simulink model "forward_inverse"  (R2023a)
settings: Solver=VariableStepAuto  StartTime=0.0  StopTime=1  RelTol=1e-3
settings Model: Creator=jeffk  LastModifiedBy=mluser
settings OptimizationCC: ReuseModelBlockBuffer=off

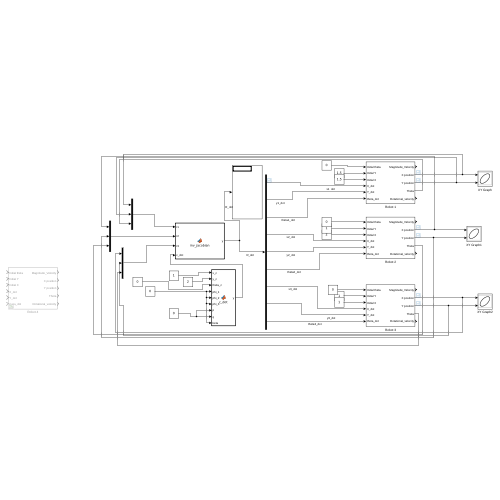
[thumbnail: Simulink's stored preview of the top-level diagram]
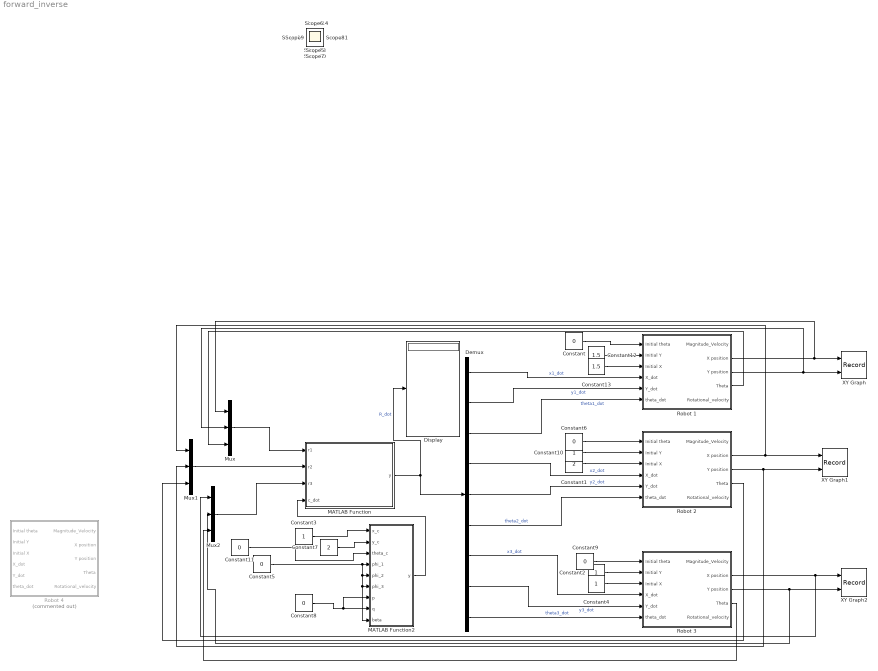
== system forward_inverse ==
  Constant{,5..6,8..9,11} (6 alike) : Constant  Value=0
  Constant1 : Constant  Value=2
  Constant{2..4,10} (4 alike) : Constant
  Constant12 : Constant  Value=1.5
  Constant13 : Constant  Value=1.5
  Constant7 : Constant  Value=2
  Demux : Demux  Outputs=9
  Display : Display
  MATLAB Function : MATLAB Function  TreatAsAtomicUnit=on
  MATLAB Function2 : MATLAB Function  TreatAsAtomicUnit=on
  Mux : Mux  Inputs=3
  Mux1 : Mux  Inputs=3
  Mux2 : Mux  Inputs=3
  Robot 1 : Subsystem
  Robot 2 : Subsystem
  Robot 3 : Subsystem
  Robot 4 : Subsystem  Commented=on
  XY Graph : Record  VariableName=robot1xy  RecordToWorkspace=on  FileSettingsInternal="{\"entries\":[{\"content\":{\"excelSettings\":{\"content\":{},\"type\":\"Streamout.ExcelSettings\"}},\"type\":\"Streamout.FileSettingStorage\",\"uuid\":\"\"}],\"packageUris\":[\"http:\\/\\/schema.mathworks.com\\/mf0\\/streamout_blocks\\/R2020a\"],\"version\":\"1.0\"}"  Layout=[1 1]  SignalsInternal="{\"entries\":[{\"content\":{\"signals\":[{\"content\":{\"blockPath\":[],\"dimensions\":[1,1],\"domain\":\"\",\"lineColor\":\"#a2142f\",\"plots\":[1],\"port\":1,\"signalID\":51,\"signalName\":\"Robot 1:2\"},\"type\":\"RecordBlkView.Signal\",\"uuid\":\"\"},{\"content\":{\"blockPath\":[],\"dimensions\":[1,1],\"domain\":\"\",\"lineColor\":\"#139fff\",\"plots\":[1],\"port\":2,\"signalID\":54,\"signalName\":\"Robot 1:3\"},\"type\":\"RecordBlkView.Signal\",\"uuid\":\"\"}]},\"type\":\"RecordBlkView.InputSignals\",\"uuid\":\"\"}],\"packageUris\":[\"http:\\/\\/schema.mathworks.com\\/mf0\\/streamout_blocks\\/R2020a\"],\"version\":\"1.0\"}"  VisualizationBindings="{\"xyplotplugin\":{\"info\":[{\"series\":[{\"bindingParametersList\":[{\"parameter\":\"X-Axis\",\"signalID\":51,\"signalName\":\"Robot 1:2\"},{\"parameter\":\"Y-Axis\",\"signalID\":54,\"signalName\":\"Robot 1:3\"}],\"seriesID\":6107}],\"subplotID\":1}]}}"  CompatibilityTag=XY
  XY Graph1 : Record  VariableName=robot2xy  RecordToWorkspace=on  FileSettingsInternal="{\"entries\":[{\"content\":{\"excelSettings\":{\"content\":{},\"type\":\"Streamout.ExcelSettings\"}},\"type\":\"Streamout.FileSettingStorage\",\"uuid\":\"\"}],\"packageUris\":[\"http:\\/\\/schema.mathworks.com\\/mf0\\/streamout_blocks\\/R2020a\"],\"version\":\"1.0\"}"  Layout=[1 1]  SignalsInternal="{\"entries\":[{\"content\":{\"signals\":[{\"content\":{\"blockPath\":[],\"dimensions\":[1,1],\"domain\":\"\",\"lineColor\":\"#a2142f\",\"plots\":[1],\"port\":1,\"signalID\":35,\"signalName\":\"Robot 2:2\"},\"type\":\"RecordBlkView.Signal\",\"uuid\":\"\"},{\"content\":{\"blockPath\":[],\"dimensions\":[1,1],\"domain\":\"\",\"lineColor\":\"#139fff\",\"plots\":[1],\"port\":2,\"signalID\":38,\"signalName\":\"Robot 2:3\"},\"type\":\"RecordBlkView.Signal\",\"uuid\":\"\"}]},\"type\":\"RecordBlkView.InputSignals\",\"uuid\":\"\"}],\"packageUris\":[\"http:\\/\\/schema.mathworks.com\\/mf0\\/streamout_blocks\\/R2020a\"],\"version\":\"1.0\"}"  VisualizationBindings="{\"xyplotplugin\":{\"info\":[{\"series\":[{\"bindingParametersList\":[{\"parameter\":\"X-Axis\",\"signalID\":35,\"signalName\":\"Robot 2:2\"},{\"parameter\":\"Y-Axis\",\"signalID\":38,\"signalName\":\"Robot 2:3\"}],\"seriesID\":14312}],\"subplotID\":1}]}}"  CompatibilityTag=XY
  XY Graph2 : Record  VariableName=robot3xy  RecordToWorkspace=on  FileSettingsInternal="{\"entries\":[{\"content\":{\"excelSettings\":{\"content\":{},\"type\":\"Streamout.ExcelSettings\"}},\"type\":\"Streamout.FileSettingStorage\",\"uuid\":\"\"}],\"packageUris\":[\"http:\\/\\/schema.mathworks.com\\/mf0\\/streamout_blocks\\/R2020a\"],\"version\":\"1.0\"}"  Layout=[1 1]  SignalsInternal="{\"entries\":[{\"content\":{\"signals\":[{\"content\":{\"blockPath\":[],\"dimensions\":[1,1],\"domain\":\"\",\"lineColor\":\"#a2142f\",\"plots\":[1],\"port\":1,\"signalID\":43,\"signalName\":\"Robot 3:2\"},\"type\":\"RecordBlkView.Signal\",\"uuid\":\"\"},{\"content\":{\"blockPath\":[],\"dimensions\":[1,1],\"domain\":\"\",\"lineColor\":\"#139fff\",\"plots\":[1],\"port\":2,\"signalID\":46,\"signalName\":\"Robot 3:3\"},\"type\":\"RecordBlkView.Signal\",\"uuid\":\"\"}]},\"type\":\"RecordBlkView.InputSignals\",\"uuid\":\"\"}],\"packageUris\":[\"http:\\/\\/schema.mathworks.com\\/mf0\\/streamout_blocks\\/R2020a\"],\"version\":\"1.0\"}"  VisualizationBindings="{\"xyplotplugin\":{\"info\":[{\"series\":[{\"bindingParametersList\":[{\"parameter\":\"X-Axis\",\"signalID\":43,\"signalName\":\"Robot 3:2\"},{\"parameter\":\"Y-Axis\",\"signalID\":46,\"signalName\":\"Robot 3:3\"}],\"seriesID\":37301}],\"subplotID\":1}]}}"  CompatibilityTag=XY
  Scope{,1..14} (15 alike) : Scope
  wires:
  MATLAB Function2/1(y) -> MATLAB Function/4(c_dot)
  MATLAB Function/1(y) -> Display/1, Demux/1  "R_dot"
  Constant1/1 -> Robot 2/3(Initial X)
  Constant3/1 -> MATLAB Function2/1(x_c)
  Constant5/1 -> MATLAB Function2/9(beta), MATLAB Function2/6(phi_3), MATLAB Function2/5(phi_2), MATLAB Function2/4(phi_1)
  Robot 1/2(X position) -> Mux/1, XY Graph/1
  Demux/1 -> Robot 1/4(X_dot)  "x1_dot"
  Demux/2 -> Robot 1/5(Y_dot)  "y1_dot"
  Demux/3 -> Robot 1/6(theta_dot)  "theta1_dot"
  Demux/4 -> Robot 2/4(X_dot)  "x2_dot"
  Demux/5 -> Robot 2/5(Y_dot)  "y2_dot"
  Demux/6 -> Robot 2/6(theta_dot)  "theta2_dot"
  Robot 2/2(X position) -> Mux1/1, XY Graph1/1
  Robot 2/3(Y position) -> Mux1/2, XY Graph1/2
  Demux/7 -> Robot 3/4(X_dot)  "x3_dot"
  Demux/8 -> Robot 3/5(Y_dot)  "y3_dot"
  Demux/9 -> Robot 3/6(theta_dot)  "theta3_dot"
  Robot 3/3(Y position) -> Mux2/2, XY Graph2/2
  Robot 3/2(X position) -> Mux2/1, XY Graph2/1
  Constant7/1 -> MATLAB Function2/2(y_c)
  Constant8/1 -> MATLAB Function2/7(p), MATLAB Function2/8(q)
  Constant10/1 -> Robot 2/2(Initial Y)
  Constant11/1 -> MATLAB Function2/3(theta_c)
  Constant12/1 -> Robot 1/2(Initial Y)
  Constant13/1 -> Robot 1/3(Initial X)
  Robot 1/3(Y position) -> Mux/2, XY Graph/2
  Robot 1/4(Theta) -> Mux/3
  Mux/1 -> MATLAB Function/1(r1)
  Mux1/1 -> MATLAB Function/2(r2)
  Robot 2/4(Theta) -> Mux1/3
  Mux2/1 -> MATLAB Function/3(r3)
  Robot 3/4(Theta) -> Mux2/3
  Constant2/1 -> Robot 3/2(Initial Y)
  Constant4/1 -> Robot 3/3(Initial X)
  Constant/1 -> Robot 1/1(Initial theta)
  Constant6/1 -> Robot 2/1(Initial theta)
  Constant9/1 -> Robot 3/1(Initial theta)

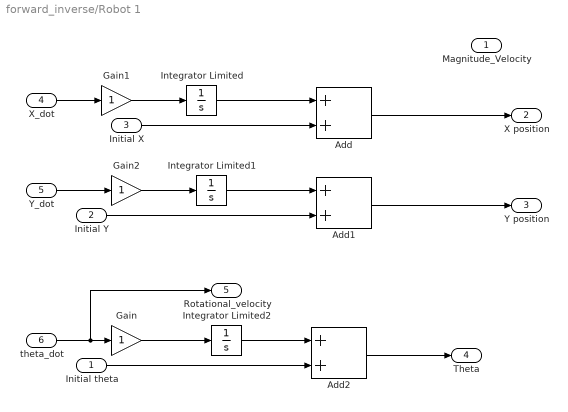
== system forward_inverse/Robot 1 ==
  Initial theta : Inport
  Initial Y : Inport  Port=2
  Initial X : Inport  Port=3
  X_dot : Inport  Port=4
  Y_dot : Inport  Port=5
  theta_dot : Inport  Port=6
  Add : Sum
  Add1 : Sum
  Add2 : Sum
  Gain : Gain
  Gain1 : Gain
  Gain2 : Gain
  Integrator Limited : Integrator  LimitOutput=on
  Integrator Limited1 : Integrator  LimitOutput=on
  Integrator Limited2 : Integrator  LimitOutput=on
  Magnitude_Velocity : Outport
  X position : Outport  Port=2
  Y position : Outport  Port=3
  Theta : Outport  Port=4
  Rotational_velocity : Outport  Port=5
  wires:
  theta_dot/1 -> Rotational_velocity/1, Gain/1
  Add1/1 -> Y position/1
  Add2/1 -> Theta/1
  Initial Y/1 -> Add1/2
  Initial X/1 -> Add/2
  Gain/1 -> Integrator Limited2/1
  X_dot/1 -> Gain1/1
  Integrator Limited/1 -> Add/1
  Y_dot/1 -> Gain2/1
  Initial theta/1 -> Add2/2
  Add/1 -> X position/1
  Gain1/1 -> Integrator Limited/1
  Integrator Limited1/1 -> Add1/1
  Gain2/1 -> Integrator Limited1/1
  Integrator Limited2/1 -> Add2/1

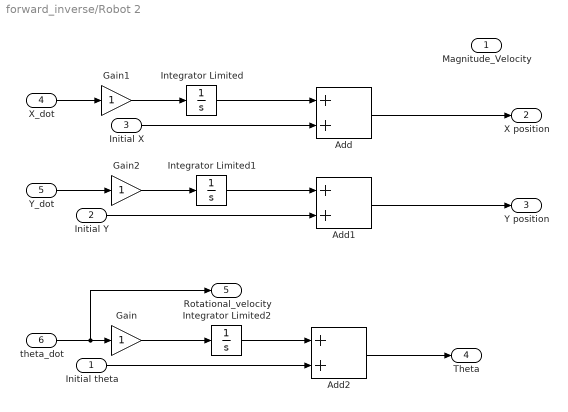
== system forward_inverse/Robot 2 ==
  Initial theta : Inport
  Initial Y : Inport  Port=2
  Initial X : Inport  Port=3
  X_dot : Inport  Port=4
  Y_dot : Inport  Port=5
  theta_dot : Inport  Port=6
  Add : Sum
  Add1 : Sum
  Add2 : Sum
  Gain : Gain
  Gain1 : Gain
  Gain2 : Gain
  Integrator Limited : Integrator  LimitOutput=on
  Integrator Limited1 : Integrator  LimitOutput=on
  Integrator Limited2 : Integrator  LimitOutput=on
  Magnitude_Velocity : Outport
  X position : Outport  Port=2
  Y position : Outport  Port=3
  Theta : Outport  Port=4
  Rotational_velocity : Outport  Port=5
  wires:
  theta_dot/1 -> Rotational_velocity/1, Gain/1
  Add1/1 -> Y position/1
  Add2/1 -> Theta/1
  Initial Y/1 -> Add1/2
  Initial X/1 -> Add/2
  Gain/1 -> Integrator Limited2/1
  X_dot/1 -> Gain1/1
  Integrator Limited/1 -> Add/1
  Y_dot/1 -> Gain2/1
  Initial theta/1 -> Add2/2
  Add/1 -> X position/1
  Gain1/1 -> Integrator Limited/1
  Integrator Limited1/1 -> Add1/1
  Gain2/1 -> Integrator Limited1/1
  Integrator Limited2/1 -> Add2/1

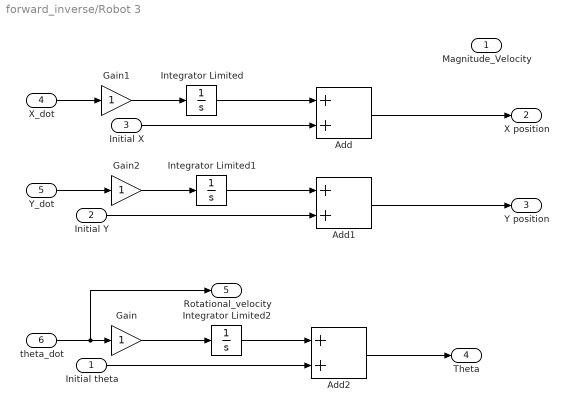
== system forward_inverse/Robot 3 ==
  Initial theta : Inport
  Initial Y : Inport  Port=2
  Initial X : Inport  Port=3
  X_dot : Inport  Port=4
  Y_dot : Inport  Port=5
  theta_dot : Inport  Port=6
  Add : Sum
  Add1 : Sum
  Add2 : Sum
  Gain : Gain
  Gain1 : Gain
  Gain2 : Gain
  Integrator Limited : Integrator  LimitOutput=on
  Integrator Limited1 : Integrator  LimitOutput=on
  Integrator Limited2 : Integrator  LimitOutput=on
  Magnitude_Velocity : Outport
  X position : Outport  Port=2
  Y position : Outport  Port=3
  Theta : Outport  Port=4
  Rotational_velocity : Outport  Port=5
  wires:
  theta_dot/1 -> Rotational_velocity/1, Gain/1
  Add1/1 -> Y position/1
  Add2/1 -> Theta/1
  Initial Y/1 -> Add1/2
  Initial X/1 -> Add/2
  Gain/1 -> Integrator Limited2/1
  X_dot/1 -> Gain1/1
  Integrator Limited/1 -> Add/1
  Y_dot/1 -> Gain2/1
  Initial theta/1 -> Add2/2
  Add/1 -> X position/1
  Gain1/1 -> Integrator Limited/1
  Integrator Limited1/1 -> Add1/1
  Gain2/1 -> Integrator Limited1/1
  Integrator Limited2/1 -> Add2/1

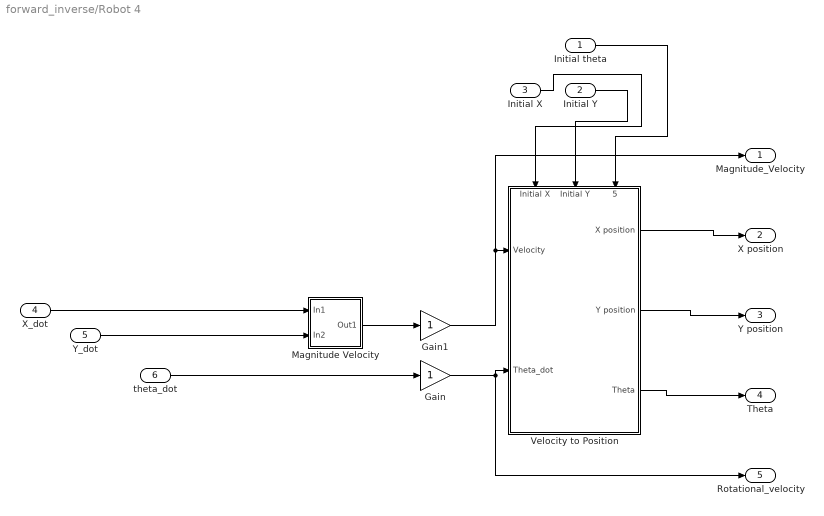
== system forward_inverse/Robot 4 ==
  Initial theta : Inport
  Initial Y : Inport  Port=2
  Initial X : Inport  Port=3
  X_dot : Inport  Port=4
  Y_dot : Inport  Port=5
  theta_dot : Inport  Port=6
  Gain : Gain
  Gain1 : Gain
  Magnitude Velocity : Subsystem
  Velocity to Position : Subsystem
      settings: PortSchema="{\"entries\":[{\"content\":{\"sides\":[{\"content\":{\"connectorIds\":[\"In1\",\"In2\"]},\"type\":\"ConnectorPlacement.EquallySpacedRectSide\",\"uuid\":\"ed42c111-3869-4678-b806-ef13090f8487\"},{\"content\":{\"connectorIds\":[\"Out1\",\"Out2\",\"Out3\"],\"side\":\"RIGHT\"},\"type\":\"ConnectorPlacement.EquallySpacedRectSide\",\"uuid\":\"c39d7e72-420d-4c07-ad85-46adecc61332\"},{\"content\":{\"connectorIds\":[\"In3\",\"In4\",\"In5\"],\"side\":\"TOP\"},\"type\":\"ConnectorPlacement.EquallySpacedRectSide\",\"uuid\":\"00432483-f433-462f-ae6c-defd83190e20\"}]},\"type\":\"ConnectorPlacement.EquallySpacedConnector\",\"uuid\":\"21f89f11-49c0-4b12-b97c-36b21e537b31\"}],\"packageUris\":[\"http://schema.mathworks.com/mf0/Connector/R2020b\"],\"version\":\"1.0\"}"
  Magnitude_Velocity : Outport
  X position : Outport  Port=2
  Y position : Outport  Port=3
  Theta : Outport  Port=4
  Rotational_velocity : Outport  Port=5
  wires:
  theta_dot/1 -> Gain/1
  Velocity to Position/2(Y position) -> Y position/1
  Velocity to Position/3(Theta) -> Theta/1
  Initial Y/1 -> Velocity to Position/4(Initial Y)
  Initial X/1 -> Velocity to Position/3(Initial X)
  Gain/1 -> Rotational_velocity/1, Velocity to Position/2(Theta_dot)
  Magnitude Velocity/1(Out1) -> Gain1/1
  Gain1/1 -> Magnitude_Velocity/1, Velocity to Position/1(Velocity)
  X_dot/1 -> Magnitude Velocity/1(In1)
  Velocity to Position/1(X position) -> X position/1
  Y_dot/1 -> Magnitude Velocity/2(In2)
  Initial theta/1 -> Velocity to Position/5(Initial theta)

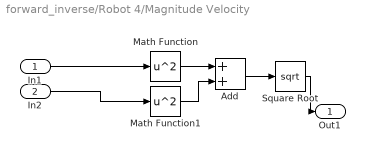
== system forward_inverse/Robot 4/Magnitude Velocity ==
  In1 : Inport
  In2 : Inport  Port=2
  Add : Sum
  Math Function : Math  Operator=square
  Math Function1 : Math  Operator=square
  Square Root : Sqrt
  Out1 : Outport
  wires:
  Math Function1/1 -> Add/2
  Add/1 -> Square Root/1
  In2/1 -> Math Function1/1
  Math Function/1 -> Add/1
  In1/1 -> Math Function/1
  Square Root/1 -> Out1/1

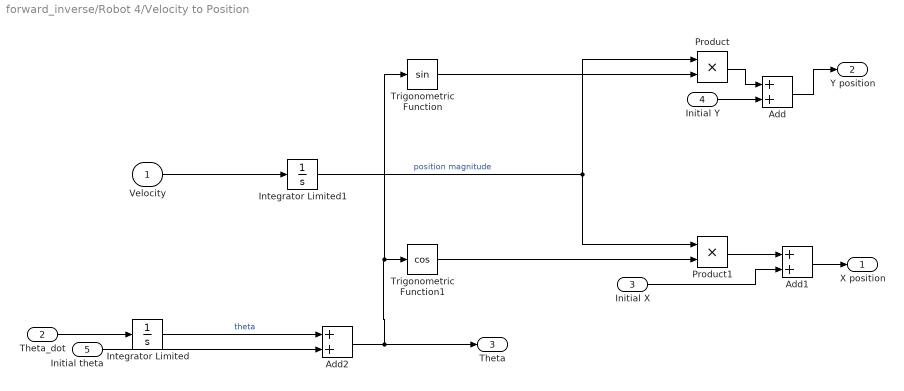
== system forward_inverse/Robot 4/Velocity to Position ==
  Velocity : Inport
  Theta_dot : Inport  Port=2
  Initial X : Inport  Port=3
  Initial Y : Inport  Port=4
  Initial theta : Inport  Port=5
  Add : Sum
  Add1 : Sum
  Add2 : Sum
  Integrator Limited : Integrator  LimitOutput=on  LowerSaturationLimit=0
  Integrator Limited1 : Integrator  LimitOutput=on  LowerSaturationLimit=0
  Product : Product
  Product1 : Product
  Trigonometric Function : Trigonometry
  Trigonometric Function1 : Trigonometry  Operator=cos
  X position : Outport
  Y position : Outport  Port=2
  Theta : Outport  Port=3
  wires:
  Trigonometric Function1/1 -> Product1/2
  Product/1 -> Add/1
  Integrator Limited/1 -> Add2/1  "theta"
  Integrator Limited1/1 -> Product/1, Product1/1  "position magnitude"
  Product1/1 -> Add1/1
  Trigonometric Function/1 -> Product/2
  Theta_dot/1 -> Integrator Limited/1
  Velocity/1 -> Integrator Limited1/1
  Initial Y/1 -> Add/2
  Add/1 -> Y position/1
  Add1/1 -> X position/1
  Initial X/1 -> Add1/2
  Initial theta/1 -> Add2/2
  Add2/1 -> Theta/1, Trigonometric Function/1, Trigonometric Function1/1

== matlab function forward_inverse/MATLAB Function ==
  data: r1 input; y output; r2 input; r3 input; c_dot input
function y = inv_jacobian(r1, r2, r3, c_dot)
% % This will be the forward Jacobian
% % the paramaters r are arrays of size three of format: [x, y, theta]
% % c_dot is the column vector of the derivative of the cluster variables
% % c_dot{1} : x_c
% % c_dot{2} : y_c
% % c_dot{3} : theta_c
% % c_dot{4} : phi_1
% % c_dot{5} : phi_2
% % c_dot{6} : phi_3
% % c_dot{7} : p
% % c_dot{8} : q
% % c_dot{9} : beta
% 
% syms x1 y1 th1 x2 y2 th2 x3 y3 th3
% 
% x_c = (x1 + x2 + x3)/3.0;
% y_c = (y1 + y2 + y3)/3.0;
% theta_c = atan2( (2.0/3.0) * x1 - (1.0/3.0) * (x2 + x3), (2.0/3.0) * y1 - (1.0/3.0) * (y2 + y3));
% phi_1 = th1 + theta_c;
% phi_2 = th2 + theta_c;
% phi_3 = th3 + theta_c;
% p = sqrt( (x1 - x2)^2 + (y1 - y2)^2);
% q = sqrt( (x3 - x1)^2 + (y3 - y1)^2);
% beta = acos( (p^2 + q^2 - (x3 - x2)^2 - (y3 - y2)^2) / (2 * p * q));
% 
% 
% F = [x_c, y_c, theta_c, phi_1, phi_2, phi_3, p, q, beta];
% X = [x1, y1, th1, x2, y2, th2, x3, y3, th3];
% 
% J = jacobian(F, X);
% J_inv = inv(J);
% 
% J_inv_with_current_values = double( subs (J_inv, [x1, y1, th1, x2, y2, th2, x3, y3, th3], [r1{1}, r1{2}, r1{3}, r2{1}, r2{2}, r2{3}, r3{1}, r3{2}, r3{3}]) );
% 
% R_dot = J_inv_with_current_values * [c_dot{1}; c_dot{2}; c_dot{3}; c_dot{4}; c_dot{5}; c_dot{6}; c_dot{7}; c_dot{8}; c_dot{9}];
coder.extrinsic("inv_jacob");
y = [0; 0; 0; 0; 0; 0; 0; 0; 0];

y = inv_jacob(r1, r2, r3, c_dot);

== matlab function forward_inverse/MATLAB Function2 ==
  data: x_c input; y output; y_c input; theta_c input; phi_1 input; phi_2 input; phi_3 input; p input; q input; beta input
function y = c_dot(x_c, y_c, theta_c, phi_1, phi_2, phi_3, p, q, beta)

y = [x_c, y_c, theta_c, phi_1, phi_2, phi_3, p, q, beta];
